simulink model "sampleModel186"  (Simulink 9.1)
settings: Solver=VariableStepAuto  StartTime=0.0  StopTime=10.0  RelTol=1e-3
undefined symbols (not defined in the file): DiscIntNeverNeededParam, Newton, Raphson
libraries: simulink x39
(part 1 of 2)
settings Model: SuppressorTable="22 serialization::archive 11 0 6 0 0 1 8 0 0 0 0 6 0 0 1 0 23 sampleModel186/cfblk100 0 6 0 0 2 8 0 0 0 0 6 41 Simulink:DataType:WarningOverFlowDetected 0 0 0 6 0  0  0 0 0 0 8 20160608 0 0 0 15 23 17 0 1 40 SimulinkFixedPoint:util:Overflowoccurred 0 0 0  0  8 20160608 0 15 23 17 0 1"  Creator=DELL  LastModifiedBy=DELL
settings DataIOCC: SaveFormat=Dataset
settings OptimizationCC: LifeSpan=auto
settings DebuggingCC: UnderspecifiedInitializationDetection=Simplified  MergeDetectMultiDrivingBlocksExec=error  SFUnexpectedBacktrackingDiag=error  SFNoUnconditionalDefaultTransitionDiag=error  SFExecutionAtInitializationDiag=warning
settings HardwareCC: ProdBitPerPointer=64  ProdBitPerSizeT=64  ProdBitPerPtrDiffT=64  ProdLargestAtomicFloat=Float  ProdIntDivRoundTo=Zero  ProdEndianess=LittleEndian  ProdWordSize=64  ProdHWDeviceType=Intel->x86-64 (Windows64)
settings ModelReferenceCC: PropagateSignalLabelsOutOfModel=on
settings CodeAppCC: StateflowObjectComments=off
settings GRTTargetCC: TargetLangStandard=C99 (ISO)  CombineOutputUpdateFcns=on  GRTInterface=off
settings ConfigComp: CovMetricSettings=dwe  CovHtmlReporting=off  CovSaveCumulativeToWorkspaceVar=off  CovSaveSingleToWorkspaceVar=off  CovExternalEMLEnable=on

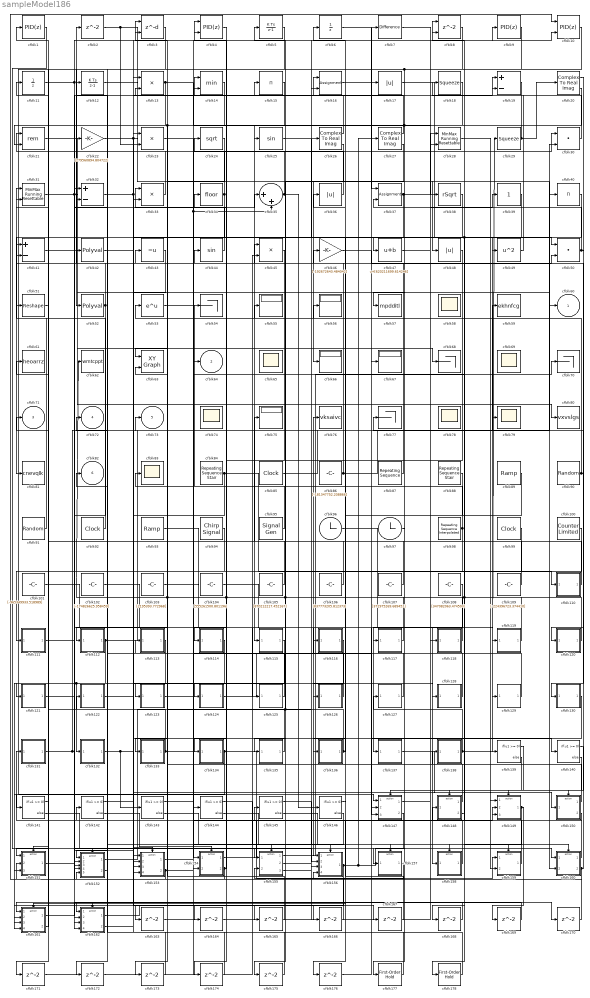
== system sampleModel186 ==
  cfblk1 : simulink/Continuous/PID Controller  Controller=PID  TimeDomain=Discrete-time  SampleTime=1  IntegratorMethod=Forward Euler  FilterMethod=Forward Euler  Form=Parallel  UseFilter=on  ControllerParametersSource=internal  P=1  I=1  D=0  N=100  InitialConditionSource=internal  InitialConditionForIntegrator=0  InitialConditionForFilter=0  ExternalReset=none  LimitOutput=off  UpperSaturationLimit=inf  LowerSaturationLimit=-inf  LinearizeAsGain=off  AntiWindupMode=none  Kb=1  TrackingMode=off  Kt=1  PParamMin=[]  PParamMax=[]  IParamMin=[]  IParamMax=[]  DParamMin=[]  DParamMax=[]  NParamMin=[]  NParamMax=[]  KbParamMin=[]  KbParamMax=[]  KtParamMin=[]  KtParamMax=[]  POutMin=[]  POutMax=[]  IOutMin=[]  IOutMax=[]  DOutMin=[]  DOutMax=[]  NOutMin=[]  NOutMax=[]  KbOutMin=[]  KbOutMax=[]  KtOutMin=[]  KtOutMax=[]  IntegratorOutMin=[]  IntegratorOutMax=[]  FilterOutMin=[]  FilterOutMax=[]  SumOutMin=[]  SumOutMax=[]  SumI1OutMin=[]  SumI1OutMax=[]  SumI2OutMin=[]  SumI2OutMax=[]  SumI3OutMin=[]  SumI3OutMax=[]  SumDOutMin=[]  SumDOutMax=[]  SaturationOutMin=[]  SaturationOutMax=[]  IntegratorContinuousStateAttributes=''  IntegratorStateMustResolveToSignalObject=off  IntegratorRTWStateStorageClass=Auto  FilterContinuousStateAttributes=''  FilterStateMustResolveToSignalObject=off  FilterRTWStateStorageClass=Auto  DifferentiatorICPrevScaledInput=0  DifferentiatorOutMin=[]  DifferentiatorOutMax=[]  FilterDiffOutCoefMin=[]  FilterDiffOutCoefMax=[]  SumDenOutMin=[]  SumDenOutMax=[]  SumNumOutMin=[]  SumNumOutMax=[]  ReciprocalOutMin=[]  ReciprocalOutMax=[]  DivideOutMin=[]  DivideOutMax=[]  TunerSelectOption=Transfer Function Based (PID Tuner App)
  cfblk10 : simulink/Continuous/PID Controller (2DOF)  Controller=PID  TimeDomain=Discrete-time  SampleTime=1  IntegratorMethod=Forward Euler  FilterMethod=Forward Euler  Form=Parallel  UseFilter=on  ControllerParametersSource=internal  P=1  I=1  D=0  N=100  b=1  c=1  InitialConditionSource=internal  InitialConditionForIntegrator=0  InitialConditionForFilter=0  ExternalReset=none  LimitOutput=off  UpperSaturationLimit=inf  LowerSaturationLimit=-inf  LinearizeAsGain=off  AntiWindupMode=none  Kb=1  TrackingMode=off  Kt=1  PParamMin=[]  PParamMax=[]  IParamMin=[]  IParamMax=[]  DParamMin=[]  DParamMax=[]  NParamMin=[]  NParamMax=[]  bParamMin=[]  bParamMax=[]  cParamMin=[]  cParamMax=[]  KbParamMin=[]  KbParamMax=[]  KtParamMin=[]  KtParamMax=[]  POutMin=[]  POutMax=[]  IOutMin=[]  IOutMax=[]  DOutMin=[]  DOutMax=[]  NOutMin=[]  NOutMax=[]  bOutMin=[]  bOutMax=[]  cOutMin=[]  cOutMax=[]  KbOutMin=[]  KbOutMax=[]  KtOutMin=[]  KtOutMax=[]  IntegratorOutMin=[]  IntegratorOutMax=[]  FilterOutMin=[]  FilterOutMax=[]  SumOutMin=[]  SumOutMax=[]  Sum1OutMin=[]  Sum1OutMax=[]  Sum2OutMin=[]  Sum2OutMax=[]  Sum3OutMin=[]  Sum3OutMax=[]  SumI1OutMin=[]  SumI1OutMax=[]  SumI2OutMin=[]  SumI2OutMax=[]  SumI3OutMin=[]  SumI3OutMax=[]  SumDOutMin=[]  SumDOutMax=[]  SaturationOutMin=[]  SaturationOutMax=[]  IntegratorContinuousStateAttributes=''  IntegratorStateMustResolveToSignalObject=off  IntegratorRTWStateStorageClass=Auto  FilterContinuousStateAttributes=''  FilterStateMustResolveToSignalObject=off  FilterRTWStateStorageClass=Auto  DifferentiatorICPrevScaledInput=0  DifferentiatorOutMin=[]  DifferentiatorOutMax=[]  FilterDiffOutCoefMin=[]  FilterDiffOutCoefMax=[]  SumDenOutMin=[]  SumDenOutMax=[]  SumNumOutMin=[]  SumNumOutMax=[]  ReciprocalOutMin=[]  ReciprocalOutMax=[]  DivideOutMin=[]  DivideOutMax=[]  TunerSelectOption=Transfer Function Based (PID Tuner App)
  cfblk100 : simulink/Sources/Counter Limited  uplimit=[470.000000]  tsamp=-1
  cfblk101 : Constant  Value=[-965349933.518989]  SampleTime=1
  cfblk102 : Constant  Value=[-174826625.958459]  SampleTime=1
  cfblk103 : Constant  Value=[2195393.772968]  SampleTime=1
  cfblk104 : Constant  Value=[555261500.801196]  SampleTime=1
  cfblk105 : Constant  Value=[870212217.452167]  SampleTime=1
  cfblk106 : Constant  Value=[837773205.812373]  SampleTime=1
  cfblk107 : Constant  Value=[371975269.689451]  SampleTime=1
  cfblk108 : Constant  Value=[347082063.474503]  SampleTime=1
  cfblk109 : Constant  Value=[-224396723.374410]  SampleTime=1
  cfblk11 : UnitDelay
  cfblk110 : Subsystem
  cfblk111 : Subsystem
  cfblk112 : Subsystem
  cfblk113 : Subsystem
  cfblk114 : Subsystem
  cfblk115 : Subsystem
  cfblk116 : Subsystem
  cfblk117 : Subsystem
  cfblk118 : Subsystem
  cfblk119 : Subsystem
  cfblk12 : DiscreteIntegrator  ICPrevOutput=DiscIntNeverNeededParam  ICPrevScaledInput=DiscIntNeverNeededParam
  cfblk120 : Subsystem
  cfblk121 : Subsystem
  cfblk122 : Subsystem
  cfblk123 : Subsystem
  cfblk124 : Subsystem
  cfblk125 : Subsystem
  cfblk126 : Subsystem
  cfblk127 : Subsystem
  cfblk128 : Subsystem
  cfblk129 : Subsystem
  cfblk13 : Product
  cfblk130 : Subsystem
  cfblk131 : Subsystem
  cfblk132 : Subsystem
  cfblk133 : Subsystem
  cfblk134 : Subsystem
  cfblk135 : Subsystem
  cfblk136 : Subsystem
  cfblk137 : Subsystem
  cfblk138 : Subsystem
  cfblk{139..146} (8 alike) : If  IfExpression=u1 >= 0  SampleTime=1
  cfblk14 : MinMax  Inputs=2
  cfblk147 : Subsystem  TreatAsAtomicUnit=on
  cfblk148 : Subsystem  TreatAsAtomicUnit=on
  cfblk149 : Subsystem  TreatAsAtomicUnit=on
  cfblk15 : Product  Inputs=*
  cfblk150 : Subsystem  TreatAsAtomicUnit=on
  cfblk151 : Subsystem  TreatAsAtomicUnit=on
  cfblk152 : Subsystem  TreatAsAtomicUnit=on
  cfblk153 : Subsystem  TreatAsAtomicUnit=on
  cfblk154 : Subsystem  TreatAsAtomicUnit=on
  cfblk155 : Subsystem  TreatAsAtomicUnit=on
  cfblk156 : Subsystem  TreatAsAtomicUnit=on
  cfblk157 : Subsystem  TreatAsAtomicUnit=on
  cfblk158 : Subsystem  TreatAsAtomicUnit=on
  cfblk159 : Subsystem  TreatAsAtomicUnit=on
  cfblk16 : Assignment  DiagnosticForDimensions=Warning  IndexOptions=Index vector (dialog)  Indices=1  OutputSizes=1
  cfblk160 : Subsystem  TreatAsAtomicUnit=on
  cfblk161 : Subsystem  TreatAsAtomicUnit=on
  cfblk162 : Subsystem  TreatAsAtomicUnit=on
  cfblk{2,163..176} (15 alike) : Delay  SampleTime=1
  cfblk17 : Abs
  cfblk177 : simulink/Discrete/First-Order Hold  DisableCoverage=on  Ts=1
      settings: SourceProductName=Simulink  SourceProductBaseCode=SL
  cfblk178 : simulink/Discrete/First-Order Hold  DisableCoverage=on  Ts=1
      settings: SourceProductName=Simulink  SourceProductBaseCode=SL
  cfblk18 : Squeeze
  cfblk19 : Sum  Inputs=+-
  cfblk20 : ComplexToRealImag
  cfblk21 : Math  Operator=rem  SaturateOnIntegerOverflow=on
  cfblk22 : Gain  Gain=[279560894.804722]
  cfblk23 : Product
  cfblk24 : Sqrt  SaturateOnIntegerOverflow=on
  cfblk25 : Trigonometry
  cfblk26 : ComplexToRealImag
  cfblk27 : ComplexToRealImag
  cfblk28 : simulink/Math Operations/MinMax Running Resettable  Function=min  vinit=0.0
  cfblk29 : Squeeze
  cfblk3 : Delay  DelayLengthSource=Input port  SampleTime=1
      settings: InputPortMap=u0,p1
  cfblk30 : DotProduct  InputSameDT=on  OutDataTypeStr=Inherit: Inherit via internal rule
  cfblk31 : simulink/Math Operations/MinMax Running Resettable  Function=min  vinit=0.0
  cfblk32 : Sum  Inputs=+-
  cfblk33 : Product  Inputs=**
  cfblk34 : Rounding
  cfblk35 : Sum  Inputs=|++
  cfblk36 : Abs
  cfblk37 : Assignment  DiagnosticForDimensions=Warning  IndexOptions=Index vector (dialog)  Indices=1  OutputSizes=1
  cfblk38 : Sqrt  Operator=rSqrt  AlgorithmType=Newton-Raphson  SaturateOnIntegerOverflow=on
  cfblk39 : simulink/Math Operations/Slider Gain  gain=1  low=0  high=2
  cfblk4 : simulink/Continuous/PID Controller (2DOF)  Controller=PID  TimeDomain=Discrete-time  SampleTime=1  IntegratorMethod=Forward Euler  FilterMethod=Forward Euler  Form=Parallel  UseFilter=on  ControllerParametersSource=internal  P=1  I=1  D=0  N=100  b=1  c=1  InitialConditionSource=internal  InitialConditionForIntegrator=0  InitialConditionForFilter=0  ExternalReset=none  LimitOutput=off  UpperSaturationLimit=inf  LowerSaturationLimit=-inf  LinearizeAsGain=off  AntiWindupMode=none  Kb=1  TrackingMode=off  Kt=1  PParamMin=[]  PParamMax=[]  IParamMin=[]  IParamMax=[]  DParamMin=[]  DParamMax=[]  NParamMin=[]  NParamMax=[]  bParamMin=[]  bParamMax=[]  cParamMin=[]  cParamMax=[]  KbParamMin=[]  KbParamMax=[]  KtParamMin=[]  KtParamMax=[]  POutMin=[]  POutMax=[]  IOutMin=[]  IOutMax=[]  DOutMin=[]  DOutMax=[]  NOutMin=[]  NOutMax=[]  bOutMin=[]  bOutMax=[]  cOutMin=[]  cOutMax=[]  KbOutMin=[]  KbOutMax=[]  KtOutMin=[]  KtOutMax=[]  IntegratorOutMin=[]  IntegratorOutMax=[]  FilterOutMin=[]  FilterOutMax=[]  SumOutMin=[]  SumOutMax=[]  Sum1OutMin=[]  Sum1OutMax=[]  Sum2OutMin=[]  Sum2OutMax=[]  Sum3OutMin=[]  Sum3OutMax=[]  SumI1OutMin=[]  SumI1OutMax=[]  SumI2OutMin=[]  SumI2OutMax=[]  SumI3OutMin=[]  SumI3OutMax=[]  SumDOutMin=[]  SumDOutMax=[]  SaturationOutMin=[]  SaturationOutMax=[]  IntegratorContinuousStateAttributes=''  IntegratorStateMustResolveToSignalObject=off  IntegratorRTWStateStorageClass=Auto  FilterContinuousStateAttributes=''  FilterStateMustResolveToSignalObject=off  FilterRTWStateStorageClass=Auto  DifferentiatorICPrevScaledInput=0  DifferentiatorOutMin=[]  DifferentiatorOutMax=[]  FilterDiffOutCoefMin=[]  FilterDiffOutCoefMax=[]  SumDenOutMin=[]  SumDenOutMax=[]  SumNumOutMin=[]  SumNumOutMax=[]  ReciprocalOutMin=[]  ReciprocalOutMax=[]  DivideOutMin=[]  DivideOutMax=[]  TunerSelectOption=Transfer Function Based (PID Tuner App)
  cfblk40 : Product  Inputs=*
  cfblk41 : Sum  Inputs=+-
  cfblk42 : Polyval  Coefs=[ +2.081618890e-019, -1.441693666e-014, +4.719686976e-010, -8.536869453e-006, +1.621573104e-001, -8.087801117e+001 ]
  cfblk43 : UnaryMinus
  cfblk44 : Trigonometry
  cfblk45 : Product  Inputs=**
  cfblk46 : Gain  Gain=[-192672643.484042]
  cfblk47 : Bias  Bias=[620211699.614246]
  cfblk48 : Abs
  cfblk49 : Math  Operator=square  SaturateOnIntegerOverflow=on
  cfblk5 : DiscreteIntegrator  ICPrevOutput=DiscIntNeverNeededParam  ICPrevScaledInput=DiscIntNeverNeededParam
  cfblk50 : DotProduct  InputSameDT=on  OutDataTypeStr=Inherit: Inherit via internal rule
  cfblk51 : Reshape
  cfblk52 : Polyval  Coefs=[ +2.081618890e-019, -1.441693666e-014, +4.719686976e-010, -8.536869453e-006, +1.621573104e-001, -8.087801117e+001 ]
  cfblk53 : Math  SaturateOnIntegerOverflow=on
  cfblk{54,68,70,77} (4 alike) : Terminator
  cfblk{55..56,66..67,75} (5 alike) : Display
  cfblk57 : ToWorkspace  VariableName=mpdditl  SaveFormat=Timeseries  SampleTime=-1
  cfblk{58,65,69,74,78..79,83} (7 alike) : Scope
      cfblk58 settings: Floating=on
      cfblk65 settings: Floating=on
      cfblk69 settings: Floating=on
      cfblk74 settings: Floating=on
      cfblk78 settings: Floating=on
  cfblk59 : ToWorkspace  VariableName=ekhnfcg  SaveFormat=Timeseries  SampleTime=-1
  cfblk6 : UnitDelay
  cfblk61 : ToWorkspace  VariableName=heoarrz  SaveFormat=Timeseries  SampleTime=-1
  cfblk62 : ToWorkspace  VariableName=wmtcppt  SaveFormat=Timeseries  SampleTime=-1
  cfblk63 : simulink/Sinks/XY Graph  xmin=-1  xmax=1  ymin=-1  ymax=1  st=-1
  cfblk7 : simulink/Discrete/Difference  ICPrevInput=0.0  OutMin=[]  OutMax=[]  OutDataTypeStr=Inherit: Inherit via back propagation  OutDataType=fixdt(1, 16)  OutScaling=2^-10  DoSatur=off
  cfblk76 : ToWorkspace  VariableName=vksaivc  SaveFormat=Timeseries  SampleTime=-1
  cfblk8 : Delay  ShowEnablePort=on  SampleTime=1
      settings: InputPortMap=u0,e6
  cfblk80 : ToWorkspace  VariableName=vxvslgs  SaveFormat=Timeseries  SampleTime=-1
  cfblk81 : ToWorkspace  VariableName=cnevqlk  SaveFormat=Timeseries  SampleTime=-1
  cfblk84 : simulink/Sources/Repeating Sequence Stair  OutValues=[-951012836.376546, -301150496.338578]  tsamp=-1  OutMin=[]  OutMax=[]  OutDataTypeStr=double  OutputDataTypeScalingMode=double  OutDataType=fixdt(0,8)  ConRadixGroup=Best Precision: Vector-wise  OutScaling=2^-12
  cfblk85 : DigitalClock
  cfblk86 : Constant  Value=[-181347752.208866]  SampleTime=1
  cfblk87 : simulink/Sources/Repeating Sequence  rep_seq_t=[0 2]  rep_seq_y=[440494450.888145, 19517650.074052]
  cfblk88 : simulink/Sources/Repeating Sequence Stair  OutValues=[252287752.212713, -649877738.569084]  tsamp=-1  OutMin=[]  OutMax=[]  OutDataTypeStr=double  OutputDataTypeScalingMode=double  OutDataType=fixdt(0,8)  ConRadixGroup=Best Precision: Vector-wise  OutScaling=2^-12
  cfblk89 : simulink/Sources/Ramp  slope=[7648.383013]  start=[49.860046]  InitialOutput=[-317458.336666]
  cfblk9 : simulink/Continuous/PID Controller  Controller=PID  TimeDomain=Discrete-time  SampleTime=1  IntegratorMethod=Forward Euler  FilterMethod=Forward Euler  Form=Parallel  UseFilter=on  ControllerParametersSource=internal  P=1  I=1  D=0  N=100  InitialConditionSource=internal  InitialConditionForIntegrator=0  InitialConditionForFilter=0  ExternalReset=none  LimitOutput=off  UpperSaturationLimit=inf  LowerSaturationLimit=-inf  LinearizeAsGain=off  AntiWindupMode=none  Kb=1  TrackingMode=off  Kt=1  PParamMin=[]  PParamMax=[]  IParamMin=[]  IParamMax=[]  DParamMin=[]  DParamMax=[]  NParamMin=[]  NParamMax=[]  KbParamMin=[]  KbParamMax=[]  KtParamMin=[]  KtParamMax=[]  POutMin=[]  POutMax=[]  IOutMin=[]  IOutMax=[]  DOutMin=[]  DOutMax=[]  NOutMin=[]  NOutMax=[]  KbOutMin=[]  KbOutMax=[]  KtOutMin=[]  KtOutMax=[]  IntegratorOutMin=[]  IntegratorOutMax=[]  FilterOutMin=[]  FilterOutMax=[]  SumOutMin=[]  SumOutMax=[]  SumI1OutMin=[]  SumI1OutMax=[]  SumI2OutMin=[]  SumI2OutMax=[]  SumI3OutMin=[]  SumI3OutMax=[]  SumDOutMin=[]  SumDOutMax=[]  SaturationOutMin=[]  SaturationOutMax=[]  IntegratorContinuousStateAttributes=''  IntegratorStateMustResolveToSignalObject=off  IntegratorRTWStateStorageClass=Auto  FilterContinuousStateAttributes=''  FilterStateMustResolveToSignalObject=off  FilterRTWStateStorageClass=Auto  DifferentiatorICPrevScaledInput=0  DifferentiatorOutMin=[]  DifferentiatorOutMax=[]  FilterDiffOutCoefMin=[]  FilterDiffOutCoefMax=[]  SumDenOutMin=[]  SumDenOutMax=[]  SumNumOutMin=[]  SumNumOutMax=[]  ReciprocalOutMin=[]  ReciprocalOutMax=[]  DivideOutMin=[]  DivideOutMax=[]  TunerSelectOption=Transfer Function Based (PID Tuner App)
  cfblk90 : RandomNumber  Mean=[38383.504717]  Variance=[46527.170956]  Seed=[481409235.000000]  SampleTime=0.1
  cfblk91 : RandomNumber  Mean=[-57930.765169]  Variance=[93296.523192]  Seed=[604567942.000000]  SampleTime=0.1
  cfblk92 : DigitalClock
  cfblk93 : simulink/Sources/Ramp  slope=[805.402797]  start=[19.130150]  InitialOutput=[280438.468677]
  cfblk94 : simulink/Sources/Chirp Signal  f1=[-292046844.976813]  T=[-444072076.223065]  f2=[-648078448.170480]
  cfblk95 : SignalGenerator  Amplitude=[-110026774.580728]
  cfblk96 : Clock
  cfblk97 : Clock
  cfblk98 : simulink/Sources/Repeating Sequence Interpolated  OutValues=[-130836063.192327, 223313554.665259, -659778868.713167, 244454041.153535, 249774118.930075]  TimeValues=[0 0.1 0.5 0.6 1].'  LookUpMeth=Use Input Nearest  tsamp=0.01  OutMin=[]  OutMax=[]  OutDataTypeStr=double  OutputDataTypeScalingMode=double  OutDataType=fixdt(0,8)  OutScaling=2^-10
  cfblk99 : DigitalClock
  cfblk60 : Outport
  cfblk64 : Outport  Port=2
  cfblk71 : Outport  Port=3
  cfblk72 : Outport  Port=4
  cfblk73 : Outport  Port=5
  cfblk82 : Outport  Port=6
  wires:
  cfblk44/1 -> cfblk33/1
  cfblk113/1(cfblk2) -> cfblk132/1(cfblk1), cfblk161/4(cfblk15)
  cfblk21/1 -> cfblk80/1
  cfblk131/1(cfblk2) -> cfblk73/1, cfblk153/4(cfblk11)
  cfblk3/1 -> cfblk147/1(cfblk1)
  cfblk40/1 -> cfblk81/1
  cfblk148/1(cfblk2) -> cfblk112/1(cfblk1)
  cfblk20/1 -> cfblk77/1
  cfblk84/1 -> cfblk110/1(cfblk1), cfblk153/3(cfblk10)
  cfblk155/1(cfblk2) -> cfblk70/1
  cfblk12/1 -> cfblk66/1
  cfblk119/1(cfblk2) -> cfblk43/1, cfblk8/2
  cfblk110/1(cfblk2) -> cfblk46/1
  cfblk96/1 -> cfblk158/1(cfblk1)
  cfblk1/1 -> cfblk159/1(cfblk1)
  cfblk138/1(cfblk2) -> cfblk29/1, cfblk127/1(cfblk1)
  cfblk95/1 -> cfblk54/1
  cfblk23/1 -> cfblk154/1(cfblk1)
  cfblk2/1 -> cfblk48/1, cfblk23/2
  cfblk18/1 -> cfblk114/1(cfblk1)
  cfblk103/1 -> cfblk156/1(cfblk1)
  cfblk109/1 -> cfblk36/1
  cfblk130/1(cfblk2) -> cfblk147/2(cfblk10)
  cfblk149/1(cfblk2) -> cfblk168/1, cfblk169/1
  cfblk41/1 -> cfblk68/1
  cfblk101/1 -> cfblk144/1
  cfblk156/1(cfblk2) -> cfblk160/1(cfblk1), cfblk27/1, cfblk161/2(cfblk13)
  cfblk24/1 -> cfblk63/1
  cfblk134/1(cfblk2) -> cfblk156/2(cfblk11), cfblk161/3(cfblk14)
  cfblk136/1(cfblk2) -> cfblk113/1(cfblk1), cfblk55/1, cfblk6/1
  cfblk114/1(cfblk2) -> cfblk124/1(cfblk1)
  cfblk17/1 -> cfblk129/1(cfblk1)
  cfblk158/1(cfblk2) -> cfblk131/1(cfblk1)
  cfblk15/1 -> cfblk115/1(cfblk1)
  cfblk34/1 -> cfblk24/1, cfblk171/1
  cfblk29/1 -> cfblk25/1, cfblk20/1
  cfblk47/1 -> cfblk39/1
  cfblk124/1(cfblk2) -> cfblk67/1
  cfblk107/1 -> cfblk75/1
  cfblk154/1(cfblk2) -> cfblk148/1(cfblk1)
  cfblk137/1(cfblk2) -> cfblk159/2(cfblk12)
  cfblk117/1(cfblk2) -> cfblk14/1, cfblk42/1
  cfblk148/2(cfblk9) -> cfblk64/1
  cfblk50/1 -> cfblk120/1(cfblk1), cfblk37/2
  cfblk108/1 -> cfblk137/1(cfblk1)
  cfblk128/1(cfblk2) -> cfblk5/1
  cfblk10/1 -> cfblk52/1
  cfblk30/1 -> cfblk18/1
  cfblk28/1 -> cfblk50/1
  cfblk120/1(cfblk2) -> cfblk62/1, cfblk63/2, cfblk45/1
  cfblk87/1 -> cfblk2/1
  cfblk99/1 -> cfblk155/1(cfblk1)
  cfblk91/1 -> cfblk31/1
  cfblk42/1 -> cfblk128/1(cfblk1)
  cfblk16/1 -> cfblk17/1
  cfblk48/1 -> cfblk135/1(cfblk1)
  cfblk39/1 -> cfblk163/1, cfblk178/1
  cfblk159/1(cfblk2) -> cfblk82/1
  cfblk115/1(cfblk2) -> cfblk123/1(cfblk1)
  cfblk160/1(cfblk2) -> cfblk138/1(cfblk1)
  cfblk6/1 -> cfblk37/1
  cfblk150/1(cfblk2) -> cfblk34/1
  cfblk94/1 -> cfblk141/1
  cfblk126/1(cfblk2) -> cfblk76/1
  cfblk102/1 -> cfblk125/1(cfblk1)
  cfblk98/1 -> cfblk111/1(cfblk1), cfblk3/2
  cfblk106/1 -> cfblk71/1
  cfblk153/1(cfblk2) -> cfblk30/1
  cfblk32/1 -> cfblk8/1, cfblk49/1
  cfblk105/1 -> cfblk51/1
  cfblk147/1(cfblk2) -> cfblk118/1(cfblk1)
  cfblk133/1(cfblk2) -> cfblk11/1, cfblk116/1(cfblk1)
  cfblk118/1(cfblk2) -> cfblk56/1
  cfblk152/1(cfblk2) -> cfblk26/1
  cfblk90/1 -> cfblk130/1(cfblk1), cfblk53/1
  cfblk51/1 -> cfblk151/1(cfblk1)
  cfblk112/1(cfblk2) -> cfblk59/1, cfblk151/3(cfblk11)
  cfblk157/1(cfblk2) -> cfblk156/4(cfblk13)
  cfblk135/1(cfblk2) -> cfblk83/1
  cfblk111/1(cfblk2) -> cfblk119/1(cfblk1)
  cfblk27/1 -> cfblk16/1
  cfblk53/1 -> cfblk19/1
  cfblk97/1 -> cfblk157/1(cfblk1)
  cfblk104/1 -> cfblk139/1
  cfblk37/1 -> cfblk149/1(cfblk1), cfblk162/3(cfblk14)
  cfblk25/1 -> cfblk47/1
  cfblk8/1 -> cfblk117/1(cfblk1), cfblk172/1
  cfblk22/1 -> cfblk60/1, cfblk140/1
  cfblk45/1 -> cfblk134/1(cfblk1)
  cfblk155/2(cfblk6) -> cfblk16/2
  cfblk31/1 -> cfblk160/2(cfblk6), cfblk15/1
  cfblk46/1 -> cfblk50/2
  cfblk43/1 -> cfblk153/2(cfblk9)
  cfblk5/1 -> cfblk41/1
  cfblk85/1 -> cfblk30/2
  cfblk35/1 -> cfblk21/1, cfblk146/1
  cfblk153/2(cfblk12) -> cfblk10/1, cfblk149/3(cfblk11)
  cfblk127/1(cfblk2) -> cfblk72/1
  cfblk155/3(cfblk7) -> cfblk10/2
  cfblk36/1 -> cfblk14/2
  cfblk9/1 -> cfblk152/1(cfblk1)
  cfblk86/1 -> cfblk40/1, cfblk1/1
  cfblk19/1 -> cfblk57/1, cfblk173/1
  cfblk14/1 -> cfblk133/1(cfblk1), cfblk121/1(cfblk1)
  cfblk100/1 -> cfblk162/2(cfblk13)
  cfblk7/1 -> cfblk38/1
  cfblk151/1(cfblk2) -> cfblk79/1
  cfblk33/1 -> cfblk22/1
  cfblk116/1(cfblk2) -> cfblk126/1(cfblk1)
  cfblk129/1(cfblk2) -> cfblk4/1
  cfblk160/2(cfblk7) -> cfblk44/1, cfblk152/5(cfblk16)
  cfblk92/1 -> cfblk31/2
  cfblk52/1 -> cfblk41/2, cfblk162/4(cfblk15)
  cfblk13/1 -> cfblk21/2, cfblk28/2
  cfblk132/1(cfblk2) -> cfblk150/1(cfblk1), cfblk143/1
  cfblk152/2(cfblk17) -> cfblk122/1(cfblk1)
  cfblk147/2(cfblk12) -> cfblk152/3(cfblk14)
  cfblk93/1 -> cfblk147/3(cfblk11)
  cfblk89/1 -> cfblk136/1(cfblk1)
  cfblk123/1(cfblk2) -> cfblk9/1, cfblk35/2
  cfblk11/1 -> cfblk152/4(cfblk15), cfblk3/1
  cfblk26/1 -> cfblk4/2
  cfblk125/1(cfblk2) -> cfblk12/1
  cfblk150/2(cfblk14) -> cfblk149/2(cfblk10)
  cfblk161/2(cfblk16) -> cfblk61/1
  cfblk162/2(cfblk16) -> cfblk33/2
  cfblk154/2(cfblk15) -> cfblk13/2, cfblk151/2(cfblk10)
  cfblk121/1(cfblk2) -> cfblk35/1
  cfblk49/1 -> cfblk19/2
  cfblk139/1 -> cfblk147/Action
  cfblk139/2 -> cfblk148/Action
  cfblk140/1 -> cfblk149/Action
  cfblk140/2 -> cfblk150/Action
  cfblk141/1 -> cfblk151/Action
  cfblk141/2 -> cfblk152/Action
  cfblk142/1 -> cfblk153/Action
  cfblk142/2 -> cfblk154/Action
  cfblk143/1 -> cfblk155/Action
  cfblk143/2 -> cfblk156/Action
  cfblk144/1 -> cfblk157/Action
  cfblk144/2 -> cfblk158/Action
  cfblk145/1 -> cfblk159/Action
  cfblk145/2 -> cfblk160/Action
  cfblk146/1 -> cfblk161/Action
  cfblk146/2 -> cfblk162/Action
  cfblk163/1 -> cfblk28/1
  cfblk4/1 -> cfblk164/1
  cfblk164/1 -> cfblk156/3(cfblk12)
  cfblk26/2 -> cfblk165/1
  cfblk165/1 -> cfblk13/1
  cfblk122/1(cfblk2) -> cfblk166/1
  cfblk166/1 -> cfblk155/2(cfblk5)
  cfblk162/1(cfblk2) -> cfblk167/1
  cfblk167/1 -> cfblk145/1
  cfblk168/1 -> cfblk162/1(cfblk1)
  cfblk169/1 -> cfblk161/1(cfblk1)
  cfblk161/1(cfblk2) -> cfblk170/1
  cfblk170/1 -> cfblk152/2(cfblk13)
  cfblk171/1 -> cfblk154/2(cfblk14)
  cfblk172/1 -> cfblk45/2
  cfblk173/1 -> cfblk23/1
  cfblk20/2 -> cfblk174/1
  cfblk174/1 -> cfblk142/1
  cfblk27/2 -> cfblk175/1
  cfblk175/1 -> cfblk153/1(cfblk1)
  cfblk38/1 -> cfblk176/1
  cfblk176/1 -> cfblk7/1
  cfblk88/1 -> cfblk177/1
  cfblk177/1 -> cfblk32/1
  cfblk178/1 -> cfblk32/2

== system sampleModel186/cfblk110 ==
  cfblk1 : Inport
  cfblk2 : Outport
  wires:
  cfblk1/1 -> cfblk2/1

== system sampleModel186/cfblk111 ==
  cfblk1 : Inport
  cfblk2 : Outport
  wires:
  cfblk1/1 -> cfblk2/1

== system sampleModel186/cfblk112 ==
  cfblk1 : Inport
  cfblk2 : Outport
  wires:
  cfblk1/1 -> cfblk2/1

== system sampleModel186/cfblk113 ==
  cfblk1 : Inport
  cfblk2 : Outport
  wires:
  cfblk1/1 -> cfblk2/1

== system sampleModel186/cfblk114 ==
  cfblk1 : Inport
  cfblk2 : Outport
  wires:
  cfblk1/1 -> cfblk2/1

== system sampleModel186/cfblk115 ==
  cfblk1 : Inport
  cfblk2 : Outport
  wires:
  cfblk1/1 -> cfblk2/1

== system sampleModel186/cfblk116 ==
  cfblk1 : Inport
  cfblk2 : Outport
  wires:
  cfblk1/1 -> cfblk2/1

== system sampleModel186/cfblk117 ==
  cfblk1 : Inport
  cfblk2 : Outport
  wires:
  cfblk1/1 -> cfblk2/1

== system sampleModel186/cfblk118 ==
  cfblk1 : Inport
  cfblk2 : Outport
  wires:
  cfblk1/1 -> cfblk2/1

== system sampleModel186/cfblk119 ==
  cfblk1 : Inport
  cfblk2 : Outport
  wires:
  cfblk1/1 -> cfblk2/1

== system sampleModel186/cfblk120 ==
  cfblk1 : Inport
  cfblk2 : Outport
  wires:
  cfblk1/1 -> cfblk2/1

== system sampleModel186/cfblk121 ==
  cfblk1 : Inport
  cfblk2 : Outport
  wires:
  cfblk1/1 -> cfblk2/1

== system sampleModel186/cfblk122 ==
  cfblk1 : Inport
  cfblk2 : Outport
  wires:
  cfblk1/1 -> cfblk2/1

== system sampleModel186/cfblk123 ==
  cfblk1 : Inport
  cfblk2 : Outport
  wires:
  cfblk1/1 -> cfblk2/1

== system sampleModel186/cfblk124 ==
  cfblk1 : Inport
  cfblk2 : Outport
  wires:
  cfblk1/1 -> cfblk2/1

== system sampleModel186/cfblk125 ==
  cfblk1 : Inport
  cfblk2 : Outport
  wires:
  cfblk1/1 -> cfblk2/1

== system sampleModel186/cfblk126 ==
  cfblk1 : Inport
  cfblk2 : Outport
  wires:
  cfblk1/1 -> cfblk2/1

== system sampleModel186/cfblk127 ==
  cfblk1 : Inport
  cfblk2 : Outport
  wires:
  cfblk1/1 -> cfblk2/1

== system sampleModel186/cfblk128 ==
  cfblk1 : Inport
  cfblk2 : Outport
  wires:
  cfblk1/1 -> cfblk2/1

== system sampleModel186/cfblk129 ==
  cfblk1 : Inport
  cfblk2 : Outport
  wires:
  cfblk1/1 -> cfblk2/1

== system sampleModel186/cfblk130 ==
  cfblk1 : Inport
  cfblk2 : Outport
  wires:
  cfblk1/1 -> cfblk2/1

== system sampleModel186/cfblk131 ==
  cfblk1 : Inport
  cfblk2 : Outport
  wires:
  cfblk1/1 -> cfblk2/1

== system sampleModel186/cfblk132 ==
  cfblk1 : Inport
  cfblk2 : Outport
  wires:
  cfblk1/1 -> cfblk2/1

== system sampleModel186/cfblk133 ==
  cfblk1 : Inport
  cfblk2 : Outport
  wires:
  cfblk1/1 -> cfblk2/1

== system sampleModel186/cfblk134 ==
  cfblk1 : Inport
  cfblk2 : Outport
  wires:
  cfblk1/1 -> cfblk2/1

== system sampleModel186/cfblk135 ==
  cfblk1 : Inport
  cfblk2 : Outport
  wires:
  cfblk1/1 -> cfblk2/1

== system sampleModel186/cfblk136 ==
  cfblk1 : Inport
  cfblk2 : Outport
  wires:
  cfblk1/1 -> cfblk2/1

== system sampleModel186/cfblk137 ==
  cfblk1 : Inport
  cfblk2 : Outport
  wires:
  cfblk1/1 -> cfblk2/1

== system sampleModel186/cfblk138 ==
  cfblk1 : Inport
  cfblk2 : Outport
  wires:
  cfblk1/1 -> cfblk2/1

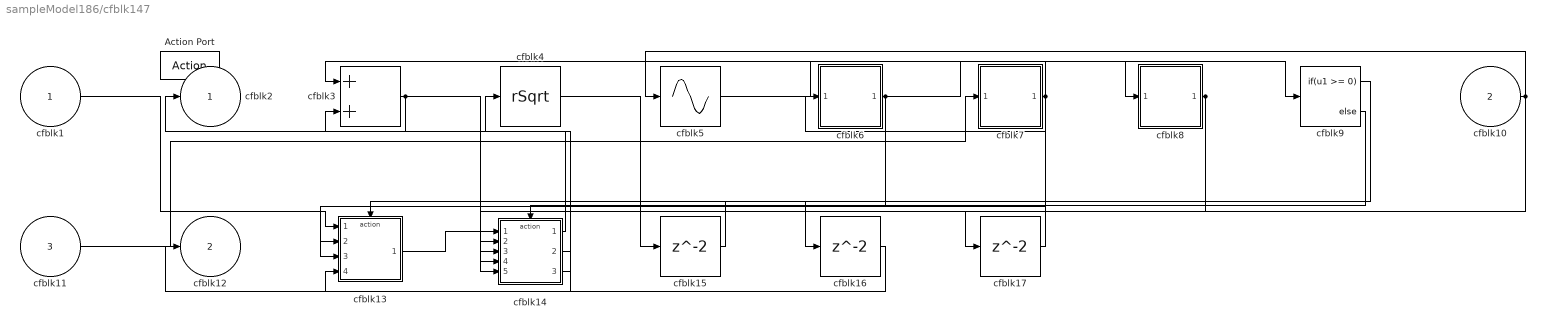
== system sampleModel186/cfblk147 ==
  cfblk1 : Inport
  cfblk10 : Inport  Port=2
  cfblk11 : Inport  Port=3
  Action Port : ActionPort  ActionType=then
  cfblk13 : Subsystem  TreatAsAtomicUnit=on
  cfblk14 : Subsystem  TreatAsAtomicUnit=on
  cfblk15 : Delay
  cfblk16 : Delay
  cfblk17 : Delay
  cfblk3 : Sum
  cfblk4 : Sqrt  Operator=rSqrt  AlgorithmType=Newton-Raphson  SaturateOnIntegerOverflow=on
  cfblk5 : Sin  TimeSource=Use external signal  SampleTime=0
  cfblk6 : Subsystem
  cfblk7 : Subsystem
  cfblk8 : Subsystem
  cfblk9 : If  IfExpression=u1 >= 0  SampleTime=1
  cfblk2 : Outport
  cfblk12 : Outport  Port=2
  wires:
  cfblk3/1 -> cfblk2/1, cfblk16/1
  cfblk11/1 -> cfblk7/1(cfblk1)
  cfblk5/1 -> cfblk9/1
  cfblk6/1(cfblk2) -> cfblk8/1(cfblk1), cfblk13/2(cfblk8)
  cfblk10/1 -> cfblk5/1, cfblk14/3(cfblk10)
  cfblk13/1(cfblk2) -> cfblk14/1(cfblk1)
  cfblk8/1(cfblk2) -> cfblk14/4(cfblk11), cfblk17/1
  cfblk7/1(cfblk2) -> cfblk3/1, cfblk13/3(cfblk9), cfblk14/5(cfblk12)
  cfblk14/1(cfblk2) -> cfblk4/1
  cfblk14/2(cfblk13) -> cfblk12/1
  cfblk14/3(cfblk14) -> cfblk3/2
  cfblk1/1 -> cfblk13/1(cfblk1)
  cfblk9/1 -> cfblk13/Action
  cfblk9/2 -> cfblk14/Action
  cfblk4/1 -> cfblk15/1
  cfblk15/1 -> cfblk14/2(cfblk9)
  cfblk16/1 -> cfblk13/4(cfblk10)
  cfblk17/1 -> cfblk6/1(cfblk1)

== system sampleModel186/cfblk148 ==
  cfblk1 : Inport
  Action Port : ActionPort  ActionType=else
  cfblk10 : Delay
  cfblk3 : Assignment  DiagnosticForDimensions=Warning  IndexOptions=Index vector (dialog)  Indices=1  OutputSizes=1
  cfblk4 : Assignment  DiagnosticForDimensions=Warning  IndexOptions=Index vector (dialog)  Indices=1  OutputSizes=1
  cfblk5 : Gain  Gain=[101234097.543843]
  cfblk6 : Subsystem
  cfblk7 : Subsystem
  cfblk8 : Subsystem
  cfblk2 : Outport
  cfblk9 : Outport  Port=2
  wires:
  cfblk6/1(cfblk2) -> cfblk4/1
  cfblk7/1(cfblk2) -> cfblk8/1(cfblk1)
  cfblk1/1 -> cfblk6/1(cfblk1)
  cfblk5/1 -> cfblk4/2, cfblk7/1(cfblk1), cfblk3/2
  cfblk3/1 -> cfblk2/1
  cfblk8/1(cfblk2) -> cfblk3/1, cfblk10/1
  cfblk4/1 -> cfblk9/1
  cfblk10/1 -> cfblk5/1

== system sampleModel186/cfblk149 ==
  cfblk1 : Inport
  cfblk10 : Inport  Port=2
  cfblk11 : Inport  Port=3
  Action Port : ActionPort  ActionType=then
  cfblk3 : simulink/Discrete/Difference  ICPrevInput=0.0  OutMin=[]  OutMax=[]  OutDataTypeStr=Inherit: Inherit via back propagation  OutDataType=fixdt(1, 16)  OutScaling=2^-10  DoSatur=off
  cfblk4 : DiscreteFilter
  cfblk5 : simulink/Math Operations/Slider Gain  gain=1  low=0  high=2
  cfblk6 : Product
  cfblk7 : Product  Inputs=**
  cfblk8 : Constant  Value=[763231843.033277]  SampleTime=1
  cfblk9 : Subsystem
  cfblk2 : Outport
  wires:
  cfblk10/1 -> cfblk9/1(cfblk1)
  cfblk4/1 -> cfblk7/1
  cfblk8/1 -> cfblk3/1
  cfblk5/1 -> cfblk7/2
  cfblk9/1(cfblk2) -> cfblk4/1
  cfblk3/1 -> cfblk5/1
  cfblk11/1 -> cfblk2/1
  cfblk1/1 -> cfblk6/1
  cfblk7/1 -> cfblk6/2

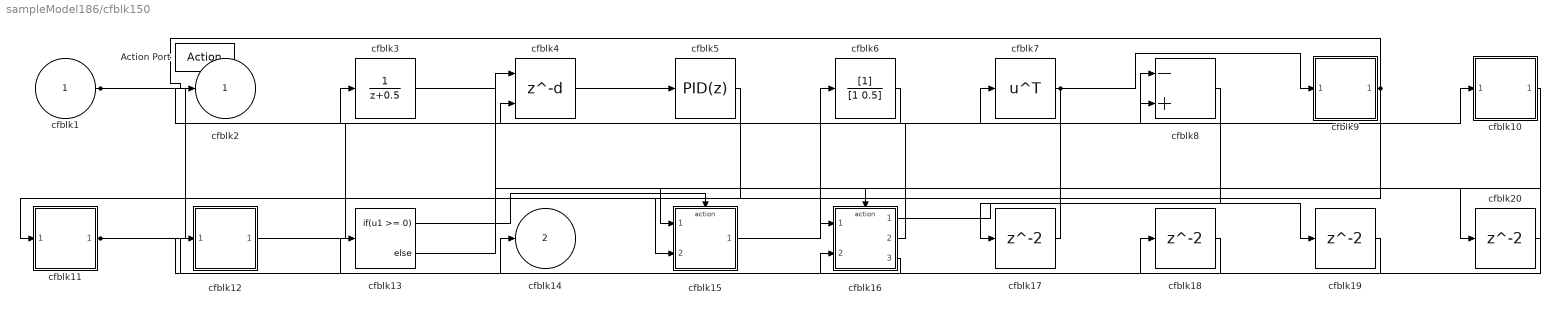
== system sampleModel186/cfblk150 ==
  cfblk1 : Inport
  Action Port : ActionPort  ActionType=else
  cfblk10 : Subsystem
  cfblk11 : Subsystem
  cfblk12 : Subsystem
  cfblk13 : If  IfExpression=u1 >= 0  SampleTime=1
  cfblk15 : Subsystem  TreatAsAtomicUnit=on
  cfblk16 : Subsystem  TreatAsAtomicUnit=on
  cfblk{17..20} (4 alike) : Delay
  cfblk3 : DiscreteTransferFcn
  cfblk4 : Delay  DelayLengthSource=Input port
      settings: InputPortMap=u0,p1
  cfblk5 : simulink/Continuous/PID Controller  Controller=PID  TimeDomain=Discrete-time  SampleTime=-1  IntegratorMethod=Forward Euler  FilterMethod=Forward Euler  Form=Parallel  UseFilter=on  ControllerParametersSource=internal  P=1  I=1  D=0  N=100  InitialConditionSource=internal  InitialConditionForIntegrator=0  InitialConditionForFilter=0  ExternalReset=none  LimitOutput=off  UpperSaturationLimit=inf  LowerSaturationLimit=-inf  LinearizeAsGain=off  AntiWindupMode=none  Kb=1  TrackingMode=off  Kt=1  PParamMin=[]  PParamMax=[]  IParamMin=[]  IParamMax=[]  DParamMin=[]  DParamMax=[]  NParamMin=[]  NParamMax=[]  KbParamMin=[]  KbParamMax=[]  KtParamMin=[]  KtParamMax=[]  POutMin=[]  POutMax=[]  IOutMin=[]  IOutMax=[]  DOutMin=[]  DOutMax=[]  NOutMin=[]  NOutMax=[]  KbOutMin=[]  KbOutMax=[]  KtOutMin=[]  KtOutMax=[]  IntegratorOutMin=[]  IntegratorOutMax=[]  FilterOutMin=[]  FilterOutMax=[]  SumOutMin=[]  SumOutMax=[]  SumI1OutMin=[]  SumI1OutMax=[]  SumI2OutMin=[]  SumI2OutMax=[]  SumI3OutMin=[]  SumI3OutMax=[]  SumDOutMin=[]  SumDOutMax=[]  SaturationOutMin=[]  SaturationOutMax=[]  IntegratorContinuousStateAttributes=''  IntegratorStateMustResolveToSignalObject=off  IntegratorRTWStateStorageClass=Auto  FilterContinuousStateAttributes=''  FilterStateMustResolveToSignalObject=off  FilterRTWStateStorageClass=Auto  DifferentiatorICPrevScaledInput=0  DifferentiatorOutMin=[]  DifferentiatorOutMax=[]  FilterDiffOutCoefMin=[]  FilterDiffOutCoefMax=[]  SumDenOutMin=[]  SumDenOutMax=[]  SumNumOutMin=[]  SumNumOutMax=[]  ReciprocalOutMin=[]  ReciprocalOutMax=[]  DivideOutMin=[]  DivideOutMax=[]  TunerSelectOption=Transfer Function Based (PID Tuner App)
  cfblk6 : DiscreteFilter
  cfblk7 : Math  Operator=transpose  SaturateOnIntegerOverflow=on
  cfblk8 : Sum  Inputs=-+
  cfblk9 : Subsystem
  cfblk2 : Outport
  cfblk14 : Outport  Port=2
  wires:
  cfblk11/1(cfblk2) -> cfblk8/1, cfblk18/1
  cfblk12/1(cfblk2) -> cfblk8/2
  cfblk15/1(cfblk2) -> cfblk6/1
  cfblk4/1 -> cfblk5/1
  cfblk7/1 -> cfblk9/1(cfblk1), cfblk16/1(cfblk1)
  cfblk6/1 -> cfblk4/2
  cfblk10/1(cfblk2) -> cfblk12/1(cfblk1)
  cfblk5/1 -> cfblk11/1(cfblk1)
  cfblk1/1 -> cfblk7/1, cfblk10/1(cfblk1)
  cfblk16/2(cfblk11) -> cfblk3/1
  cfblk16/3(cfblk12) -> cfblk14/1
  cfblk9/1(cfblk2) -> cfblk2/1, cfblk15/2(cfblk15)
  cfblk13/1 -> cfblk15/Action
  cfblk13/2 -> cfblk16/Action
  cfblk8/1 -> cfblk17/1
  cfblk17/1 -> cfblk4/1
  cfblk18/1 -> cfblk16/2(cfblk10)
  cfblk16/1(cfblk2) -> cfblk19/1
  cfblk19/1 -> cfblk13/1
  cfblk3/1 -> cfblk20/1
  cfblk20/1 -> cfblk15/1(cfblk1)

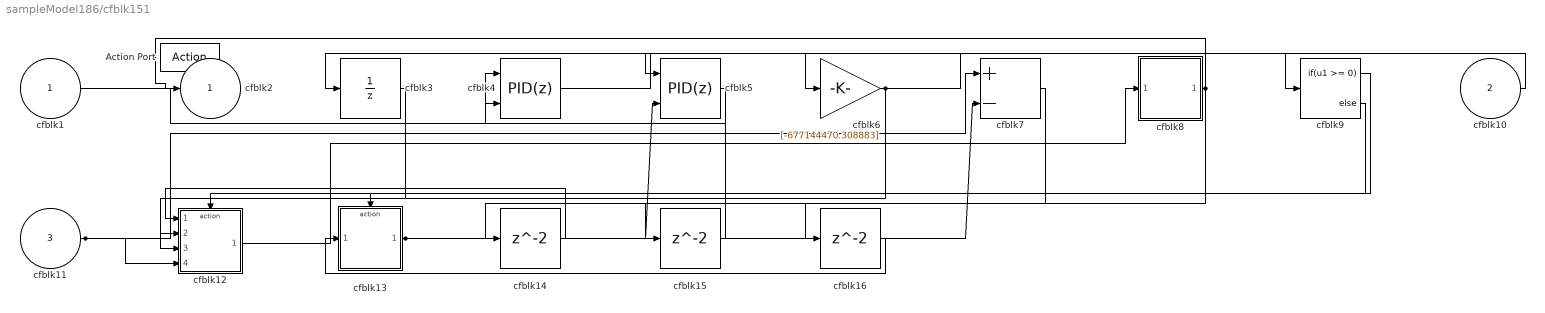
== system sampleModel186/cfblk151 ==
  cfblk1 : Inport
  cfblk10 : Inport  Port=2
  cfblk11 : Inport  Port=3
  Action Port : ActionPort  ActionType=then
  cfblk12 : Subsystem  TreatAsAtomicUnit=on
  cfblk13 : Subsystem  TreatAsAtomicUnit=on
  cfblk14 : Delay
  cfblk15 : Delay
  cfblk16 : Delay
  cfblk3 : UnitDelay  SampleTime=-1
  cfblk4 : simulink/Continuous/PID Controller (2DOF)  Controller=PID  TimeDomain=Discrete-time  SampleTime=-1  IntegratorMethod=Forward Euler  FilterMethod=Forward Euler  Form=Parallel  UseFilter=on  ControllerParametersSource=internal  P=1  I=1  D=0  N=100  b=1  c=1  InitialConditionSource=internal  InitialConditionForIntegrator=0  InitialConditionForFilter=0  ExternalReset=none  LimitOutput=off  UpperSaturationLimit=inf  LowerSaturationLimit=-inf  LinearizeAsGain=off  AntiWindupMode=none  Kb=1  TrackingMode=off  Kt=1  PParamMin=[]  PParamMax=[]  IParamMin=[]  IParamMax=[]  DParamMin=[]  DParamMax=[]  NParamMin=[]  NParamMax=[]  bParamMin=[]  bParamMax=[]  cParamMin=[]  cParamMax=[]  KbParamMin=[]  KbParamMax=[]  KtParamMin=[]  KtParamMax=[]  POutMin=[]  POutMax=[]  IOutMin=[]  IOutMax=[]  DOutMin=[]  DOutMax=[]  NOutMin=[]  NOutMax=[]  bOutMin=[]  bOutMax=[]  cOutMin=[]  cOutMax=[]  KbOutMin=[]  KbOutMax=[]  KtOutMin=[]  KtOutMax=[]  IntegratorOutMin=[]  IntegratorOutMax=[]  FilterOutMin=[]  FilterOutMax=[]  SumOutMin=[]  SumOutMax=[]  Sum1OutMin=[]  Sum1OutMax=[]  Sum2OutMin=[]  Sum2OutMax=[]  Sum3OutMin=[]  Sum3OutMax=[]  SumI1OutMin=[]  SumI1OutMax=[]  SumI2OutMin=[]  SumI2OutMax=[]  SumI3OutMin=[]  SumI3OutMax=[]  SumDOutMin=[]  SumDOutMax=[]  SaturationOutMin=[]  SaturationOutMax=[]  IntegratorContinuousStateAttributes=''  IntegratorStateMustResolveToSignalObject=off  IntegratorRTWStateStorageClass=Auto  FilterContinuousStateAttributes=''  FilterStateMustResolveToSignalObject=off  FilterRTWStateStorageClass=Auto  DifferentiatorICPrevScaledInput=0  DifferentiatorOutMin=[]  DifferentiatorOutMax=[]  FilterDiffOutCoefMin=[]  FilterDiffOutCoefMax=[]  SumDenOutMin=[]  SumDenOutMax=[]  SumNumOutMin=[]  SumNumOutMax=[]  ReciprocalOutMin=[]  ReciprocalOutMax=[]  DivideOutMin=[]  DivideOutMax=[]  TunerSelectOption=Transfer Function Based (PID Tuner App)
  cfblk5 : simulink/Continuous/PID Controller (2DOF)  Controller=PID  TimeDomain=Discrete-time  SampleTime=-1  IntegratorMethod=Forward Euler  FilterMethod=Forward Euler  Form=Parallel  UseFilter=on  ControllerParametersSource=internal  P=1  I=1  D=0  N=100  b=1  c=1  InitialConditionSource=internal  InitialConditionForIntegrator=0  InitialConditionForFilter=0  ExternalReset=none  LimitOutput=off  UpperSaturationLimit=inf  LowerSaturationLimit=-inf  LinearizeAsGain=off  AntiWindupMode=none  Kb=1  TrackingMode=off  Kt=1  PParamMin=[]  PParamMax=[]  IParamMin=[]  IParamMax=[]  DParamMin=[]  DParamMax=[]  NParamMin=[]  NParamMax=[]  bParamMin=[]  bParamMax=[]  cParamMin=[]  cParamMax=[]  KbParamMin=[]  KbParamMax=[]  KtParamMin=[]  KtParamMax=[]  POutMin=[]  POutMax=[]  IOutMin=[]  IOutMax=[]  DOutMin=[]  DOutMax=[]  NOutMin=[]  NOutMax=[]  bOutMin=[]  bOutMax=[]  cOutMin=[]  cOutMax=[]  KbOutMin=[]  KbOutMax=[]  KtOutMin=[]  KtOutMax=[]  IntegratorOutMin=[]  IntegratorOutMax=[]  FilterOutMin=[]  FilterOutMax=[]  SumOutMin=[]  SumOutMax=[]  Sum1OutMin=[]  Sum1OutMax=[]  Sum2OutMin=[]  Sum2OutMax=[]  Sum3OutMin=[]  Sum3OutMax=[]  SumI1OutMin=[]  SumI1OutMax=[]  SumI2OutMin=[]  SumI2OutMax=[]  SumI3OutMin=[]  SumI3OutMax=[]  SumDOutMin=[]  SumDOutMax=[]  SaturationOutMin=[]  SaturationOutMax=[]  IntegratorContinuousStateAttributes=''  IntegratorStateMustResolveToSignalObject=off  IntegratorRTWStateStorageClass=Auto  FilterContinuousStateAttributes=''  FilterStateMustResolveToSignalObject=off  FilterRTWStateStorageClass=Auto  DifferentiatorICPrevScaledInput=0  DifferentiatorOutMin=[]  DifferentiatorOutMax=[]  FilterDiffOutCoefMin=[]  FilterDiffOutCoefMax=[]  SumDenOutMin=[]  SumDenOutMax=[]  SumNumOutMin=[]  SumNumOutMax=[]  ReciprocalOutMin=[]  ReciprocalOutMax=[]  DivideOutMin=[]  DivideOutMax=[]  TunerSelectOption=Transfer Function Based (PID Tuner App)
  cfblk6 : Gain  Gain=[-677144470.308883]
  cfblk7 : Sum  Inputs=+-
  cfblk8 : Subsystem
  cfblk9 : If  IfExpression=u1 >= 0  SampleTime=1
  cfblk2 : Outport
  wires:
  cfblk1/1 -> cfblk4/1
  cfblk11/1 -> cfblk7/1, cfblk12/4(cfblk17)
  cfblk12/1(cfblk2) -> cfblk8/1(cfblk1)
  cfblk13/1(cfblk2) -> cfblk7/2, cfblk5/2
  cfblk8/1(cfblk2) -> cfblk2/1, cfblk5/1, cfblk15/1
  cfblk4/1 -> cfblk6/1
  cfblk6/1 -> cfblk9/1, cfblk12/3(cfblk16)
  cfblk3/1 -> cfblk12/2(cfblk15)
  cfblk10/1 -> cfblk3/1
  cfblk9/1 -> cfblk12/Action
  cfblk9/2 -> cfblk13/Action
  cfblk5/1 -> cfblk14/1
  cfblk14/1 -> cfblk12/1(cfblk1)
  cfblk15/1 -> cfblk4/2
  cfblk7/1 -> cfblk16/1
  cfblk16/1 -> cfblk13/1(cfblk1)

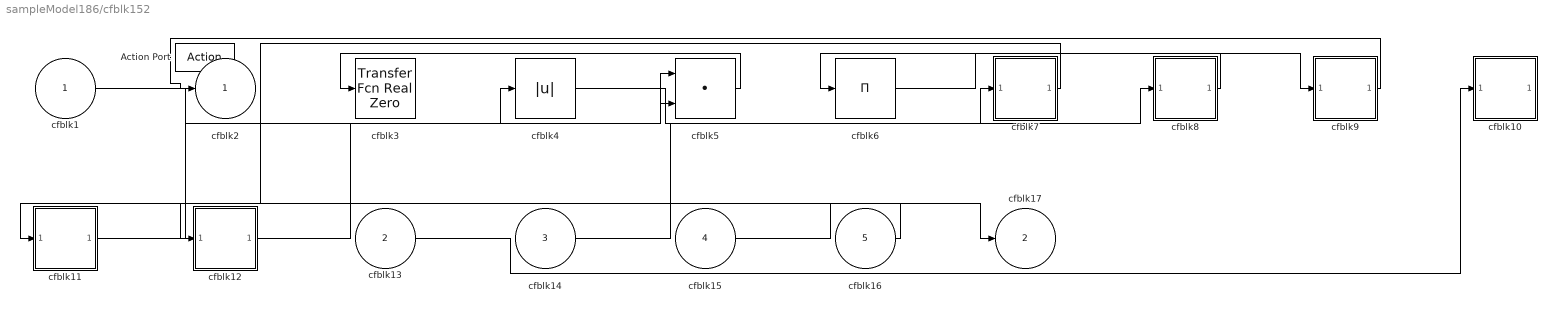
== system sampleModel186/cfblk152 ==
  cfblk1 : Inport
  cfblk13 : Inport  Port=2
  cfblk14 : Inport  Port=3
  cfblk15 : Inport  Port=4
  cfblk16 : Inport  Port=5
  Action Port : ActionPort  ActionType=else
  cfblk10 : Subsystem
  cfblk11 : Subsystem
  cfblk12 : Subsystem
  cfblk3 : simulink/Discrete/Transfer Fcn Real Zero  ZeroZ=0.75  ICPrevInput=0.0  DoSatur=off
      settings: SourceProductName=Simulink  SourceProductBaseCode=SL
  cfblk4 : Abs
  cfblk5 : DotProduct  InputSameDT=on  OutDataTypeStr=Inherit: Inherit via internal rule
  cfblk6 : Product  Inputs=*
  cfblk7 : Subsystem
  cfblk8 : Subsystem
  cfblk9 : Subsystem
  cfblk2 : Outport
  cfblk17 : Outport  Port=2
  wires:
  cfblk14/1 -> cfblk8/1(cfblk1)
  cfblk5/1 -> cfblk3/1
  cfblk7/1(cfblk2) -> cfblk11/1(cfblk1)
  cfblk12/1(cfblk2) -> cfblk5/1
  cfblk4/1 -> cfblk7/1(cfblk1)
  cfblk11/1(cfblk2) -> cfblk5/2
  cfblk13/1 -> cfblk10/1(cfblk1)
  cfblk1/1 -> cfblk4/1
  cfblk16/1 -> cfblk12/1(cfblk1)
  cfblk6/1 -> cfblk9/1(cfblk1)
  cfblk15/1 -> cfblk17/1
  cfblk9/1(cfblk2) -> cfblk2/1
  cfblk8/1(cfblk2) -> cfblk6/1

== system sampleModel186/cfblk153 ==
  cfblk1 : Inport
  cfblk9 : Inport  Port=2
  cfblk10 : Inport  Port=3
  cfblk11 : Inport  Port=4
  Action Port : ActionPort  ActionType=then
  cfblk13 : Delay
  cfblk3 : ComplexToRealImag
  cfblk4 : Subsystem
  cfblk5 : Subsystem
  cfblk6 : Subsystem
  cfblk7 : Subsystem
  cfblk8 : Subsystem
  cfblk2 : Outport
  cfblk12 : Outport  Port=2
  wires:
  cfblk10/1 -> cfblk6/1(cfblk1)
  cfblk11/1 -> cfblk5/1(cfblk1)
  cfblk8/1(cfblk2) -> cfblk2/1
  cfblk3/1 -> cfblk4/1(cfblk1)
  cfblk3/2 -> cfblk7/1(cfblk1)
  cfblk6/1(cfblk2) -> cfblk12/1
  cfblk9/1 -> cfblk8/1(cfblk1)
  cfblk7/1(cfblk2) -> cfblk13/1
  cfblk13/1 -> cfblk3/1

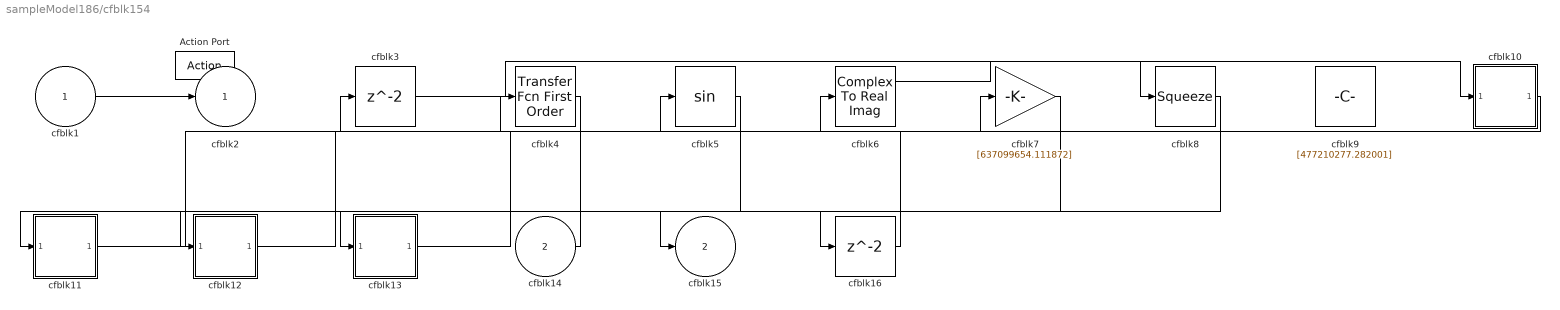
== system sampleModel186/cfblk154 ==
  cfblk1 : Inport
  cfblk14 : Inport  Port=2
  Action Port : ActionPort  ActionType=else
  cfblk10 : Subsystem
  cfblk11 : Subsystem
  cfblk12 : Subsystem
  cfblk13 : Subsystem
  cfblk16 : Delay
  cfblk3 : Delay
  cfblk4 : simulink/Discrete/Transfer Fcn First Order  PoleZ=0.95  ICPrevOutput=0.0  DoSatur=off
      settings: SourceProductName=Simulink
  cfblk5 : Trigonometry
  cfblk6 : ComplexToRealImag
  cfblk7 : Gain  Gain=[637099654.111872]
  cfblk8 : Squeeze
  cfblk9 : Constant  Value=[477210277.282001]  SampleTime=1
  cfblk2 : Outport
  cfblk15 : Outport  Port=2
  wires:
  cfblk3/1 -> cfblk8/1
  cfblk14/1 -> cfblk13/1(cfblk1)
  cfblk10/1(cfblk2) -> cfblk4/1
  cfblk4/1 -> cfblk11/1(cfblk1)
  cfblk12/1(cfblk2) -> cfblk5/1
  cfblk5/1 -> cfblk15/1
  cfblk11/1(cfblk2) -> cfblk7/1
  cfblk6/1 -> cfblk10/1(cfblk1)
  cfblk1/1 -> cfblk2/1
  cfblk13/1(cfblk2) -> cfblk6/1
  cfblk7/1 -> cfblk12/1(cfblk1)
  cfblk8/1 -> cfblk16/1
  cfblk16/1 -> cfblk3/1

== system sampleModel186/cfblk155 ==
  cfblk1 : Inport
  cfblk5 : Inport  Port=2
  Action Port : ActionPort  ActionType=then
  cfblk3 : Trigonometry
  cfblk4 : Subsystem
  cfblk2 : Outport
  cfblk6 : Outport  Port=2
  cfblk7 : Outport  Port=3
  wires:
  cfblk5/1 -> cfblk3/1, cfblk6/1
  cfblk4/1(cfblk2) -> cfblk7/1
  cfblk1/1 -> cfblk4/1(cfblk1)
  cfblk3/1 -> cfblk2/1

== system sampleModel186/cfblk156 ==
  cfblk1 : Inport
  cfblk11 : Inport  Port=2
  cfblk12 : Inport  Port=3
  cfblk13 : Inport  Port=4
  Action Port : ActionPort  ActionType=else
  cfblk10 : Subsystem
  cfblk3 : DiscreteStateSpace  SampleTime=-1
  cfblk4 : simulink/Discrete/Transfer Fcn Real Zero  ZeroZ=0.75  ICPrevInput=0.0  DoSatur=off
      settings: SourceProductName=Simulink  SourceProductBaseCode=SL
  cfblk5 : Sin  TimeSource=Use external signal  SampleTime=0
  cfblk6 : Constant  Value=[30460187.616230]  SampleTime=1
  cfblk7 : Subsystem
  cfblk8 : Subsystem
  cfblk9 : Subsystem
  cfblk2 : Outport
  wires:
  cfblk1/1 -> cfblk5/1
  cfblk4/1 -> cfblk2/1
  cfblk13/1 -> cfblk7/1(cfblk1)
  cfblk7/1(cfblk2) -> cfblk4/1
  cfblk12/1 -> cfblk10/1(cfblk1)
  cfblk6/1 -> cfblk3/1
  cfblk3/1 -> cfblk9/1(cfblk1)
  cfblk10/1(cfblk2) -> cfblk8/1(cfblk1)

== system sampleModel186/cfblk157 ==
  cfblk1 : Inport
  Action Port : ActionPort  ActionType=then
  cfblk3 : DiscreteTransferFcn
  cfblk4 : Constant  Value=[282260104.455071]  SampleTime=1
  cfblk5 : Subsystem
  cfblk6 : Subsystem
  cfblk7 : Subsystem
  cfblk2 : Outport
  wires:
  cfblk6/1(cfblk2) -> cfblk2/1
  cfblk5/1(cfblk2) -> cfblk3/1
  cfblk1/1 -> cfblk7/1(cfblk1)
  cfblk3/1 -> cfblk6/1(cfblk1)
  cfblk4/1 -> cfblk5/1(cfblk1)

== system sampleModel186/cfblk158 ==
  cfblk1 : Inport
  Action Port : ActionPort  ActionType=else
  cfblk10 : Subsystem
  cfblk11 : Subsystem
  cfblk12 : Subsystem
  cfblk13 : Delay
  cfblk3 : UnitDelay  SampleTime=-1
  cfblk4 : Sin  TimeSource=Use external signal  SampleTime=0
  cfblk5 : Sum  Inputs=+-
  cfblk6 : Constant  Value=[48957722.231244]  SampleTime=1
  cfblk7 : Constant  Value=[-200695089.141564]  SampleTime=1
  cfblk8 : Constant  Value=[-14995740.643667]  SampleTime=1
  cfblk9 : Subsystem
  cfblk2 : Outport
  wires:
  cfblk10/1(cfblk2) -> cfblk2/1
  cfblk12/1(cfblk2) -> cfblk4/1
  cfblk5/1 -> cfblk9/1(cfblk1)
  cfblk8/1 -> cfblk10/1(cfblk1)
  cfblk4/1 -> cfblk5/1
  cfblk1/1 -> cfblk11/1(cfblk1)
  cfblk11/1(cfblk2) -> cfblk12/1(cfblk1)
  cfblk6/1 -> cfblk3/1
  cfblk9/1(cfblk2) -> cfblk13/1
  cfblk13/1 -> cfblk5/2

== system sampleModel186/cfblk159 ==
  cfblk1 : Inport
  cfblk12 : Inport  Port=2
  Action Port : ActionPort  ActionType=then
  cfblk10 : Subsystem
  cfblk11 : Subsystem
  cfblk13 : Delay
  cfblk14 : Delay
  cfblk3 : simulink/Discrete/Tapped Delay  vinit=0.0  samptime=-1  NumDelays=1  DelayOrder=Oldest  includeCurrent=off
  cfblk4 : Rounding
  cfblk5 : PermuteDimensions
  cfblk6 : Sum  Inputs=+-
  cfblk7 : Assignment  DiagnosticForDimensions=Warning  IndexOptions=Index vector (dialog)  Indices=1  OutputSizes=1
  cfblk8 : Sum  Inputs=+
  cfblk9 : Subsystem
  cfblk2 : Outport
  wires:
  cfblk1/1 -> cfblk9/1(cfblk1)
  cfblk9/1(cfblk2) -> cfblk4/1
  cfblk12/1 -> cfblk2/1
  cfblk11/1(cfblk2) -> cfblk6/1
  cfblk3/1 -> cfblk7/1, cfblk7/2
  cfblk4/1 -> cfblk5/1
  cfblk6/1 -> cfblk10/1(cfblk1)
  cfblk5/1 -> cfblk8/1
  cfblk8/1 -> cfblk11/1(cfblk1)
  cfblk10/1(cfblk2) -> cfblk13/1
  cfblk13/1 -> cfblk6/2
  cfblk7/1 -> cfblk14/1
  cfblk14/1 -> cfblk3/1

== system sampleModel186/cfblk160 ==
  cfblk1 : Inport
  cfblk6 : Inport  Port=2
  Action Port : ActionPort  ActionType=else
  cfblk10 : Delay
  cfblk11 : Delay
  cfblk3 : Abs
  cfblk4 : Constant  Value=[199014671.579916]  SampleTime=1
  cfblk5 : If  IfExpression=u1 >= 0  SampleTime=1
  cfblk8 : Subsystem  TreatAsAtomicUnit=on
  cfblk9 : Subsystem  TreatAsAtomicUnit=on
  cfblk2 : Outport
  cfblk7 : Outport  Port=2
  wires:
  cfblk6/1 -> cfblk9/2(cfblk15)
  cfblk8/1(cfblk2) -> cfblk9/3(cfblk16)
  cfblk4/1 -> cfblk2/1, cfblk7/1
  cfblk1/1 -> cfblk8/1(cfblk1), cfblk8/2(cfblk12)
  cfblk8/2(cfblk13) -> cfblk3/1
  cfblk5/1 -> cfblk8/Action
  cfblk5/2 -> cfblk9/Action
  cfblk9/1(cfblk2) -> cfblk10/1
  cfblk10/1 -> cfblk5/1
  cfblk3/1 -> cfblk11/1
  cfblk11/1 -> cfblk9/1(cfblk1)

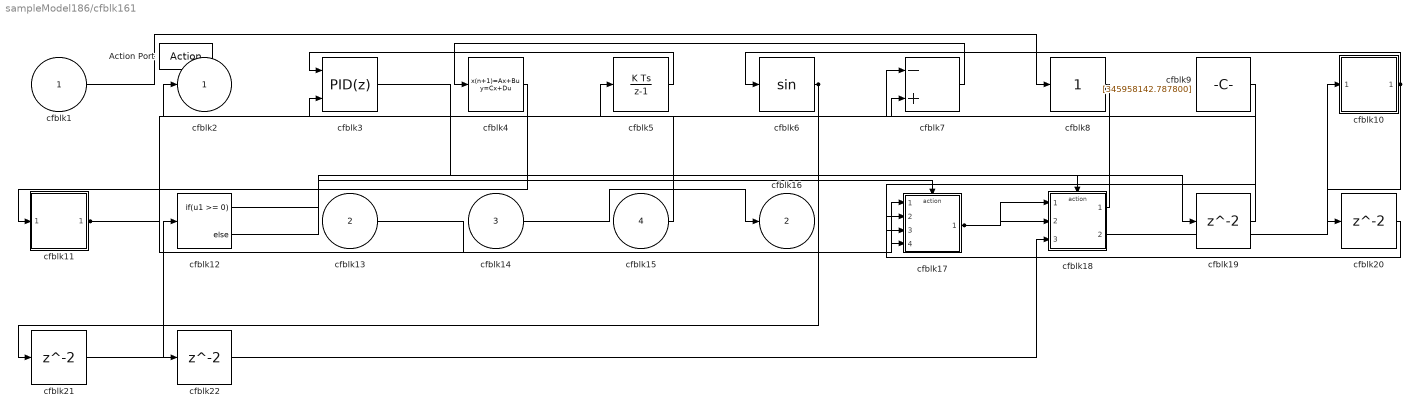
== system sampleModel186/cfblk161 ==
  cfblk1 : Inport
  cfblk13 : Inport  Port=2
  cfblk14 : Inport  Port=3
  cfblk15 : Inport  Port=4
  Action Port : ActionPort  ActionType=then
  cfblk10 : Subsystem
  cfblk11 : Subsystem
  cfblk12 : If  IfExpression=u1 >= 0  SampleTime=1
  cfblk17 : Subsystem  TreatAsAtomicUnit=on
  cfblk18 : Subsystem  TreatAsAtomicUnit=on
  cfblk{19..22} (4 alike) : Delay
  cfblk3 : simulink/Continuous/PID Controller (2DOF)  Controller=PID  TimeDomain=Discrete-time  SampleTime=-1  IntegratorMethod=Forward Euler  FilterMethod=Forward Euler  Form=Parallel  UseFilter=on  ControllerParametersSource=internal  P=1  I=1  D=0  N=100  b=1  c=1  InitialConditionSource=internal  InitialConditionForIntegrator=0  InitialConditionForFilter=0  ExternalReset=none  LimitOutput=off  UpperSaturationLimit=inf  LowerSaturationLimit=-inf  LinearizeAsGain=off  AntiWindupMode=none  Kb=1  TrackingMode=off  Kt=1  PParamMin=[]  PParamMax=[]  IParamMin=[]  IParamMax=[]  DParamMin=[]  DParamMax=[]  NParamMin=[]  NParamMax=[]  bParamMin=[]  bParamMax=[]  cParamMin=[]  cParamMax=[]  KbParamMin=[]  KbParamMax=[]  KtParamMin=[]  KtParamMax=[]  POutMin=[]  POutMax=[]  IOutMin=[]  IOutMax=[]  DOutMin=[]  DOutMax=[]  NOutMin=[]  NOutMax=[]  bOutMin=[]  bOutMax=[]  cOutMin=[]  cOutMax=[]  KbOutMin=[]  KbOutMax=[]  KtOutMin=[]  KtOutMax=[]  IntegratorOutMin=[]  IntegratorOutMax=[]  FilterOutMin=[]  FilterOutMax=[]  SumOutMin=[]  SumOutMax=[]  Sum1OutMin=[]  Sum1OutMax=[]  Sum2OutMin=[]  Sum2OutMax=[]  Sum3OutMin=[]  Sum3OutMax=[]  SumI1OutMin=[]  SumI1OutMax=[]  SumI2OutMin=[]  SumI2OutMax=[]  SumI3OutMin=[]  SumI3OutMax=[]  SumDOutMin=[]  SumDOutMax=[]  SaturationOutMin=[]  SaturationOutMax=[]  IntegratorContinuousStateAttributes=''  IntegratorStateMustResolveToSignalObject=off  IntegratorRTWStateStorageClass=Auto  FilterContinuousStateAttributes=''  FilterStateMustResolveToSignalObject=off  FilterRTWStateStorageClass=Auto  DifferentiatorICPrevScaledInput=0  DifferentiatorOutMin=[]  DifferentiatorOutMax=[]  FilterDiffOutCoefMin=[]  FilterDiffOutCoefMax=[]  SumDenOutMin=[]  SumDenOutMax=[]  SumNumOutMin=[]  SumNumOutMax=[]  ReciprocalOutMin=[]  ReciprocalOutMax=[]  DivideOutMin=[]  DivideOutMax=[]  TunerSelectOption=Transfer Function Based (PID Tuner App)
  cfblk4 : DiscreteStateSpace  SampleTime=-1
  cfblk5 : DiscreteIntegrator  SampleTime=-1  ICPrevOutput=DiscIntNeverNeededParam  ICPrevScaledInput=DiscIntNeverNeededParam
  cfblk6 : Trigonometry
  cfblk7 : Sum  Inputs=-+
  cfblk8 : simulink/Math Operations/Slider Gain  gain=1  low=0  high=2
  cfblk9 : Constant  Value=[345958142.787800]  SampleTime=1
  cfblk2 : Outport
  cfblk16 : Outport  Port=2
  wires:
  cfblk17/1(cfblk2) -> cfblk18/1(cfblk1), cfblk18/2(cfblk15)
  cfblk15/1 -> cfblk2/1
  cfblk7/1 -> cfblk4/1
  cfblk1/1 -> cfblk8/1
  cfblk13/1 -> cfblk17/1(cfblk1)
  cfblk4/1 -> cfblk11/1(cfblk1)
  cfblk18/1(cfblk2) -> cfblk5/1
  cfblk10/1(cfblk2) -> cfblk6/1, cfblk20/1
  cfblk18/2(cfblk17) -> cfblk10/1(cfblk1)
  cfblk8/1 -> cfblk7/2
  cfblk6/1 -> cfblk21/1, cfblk22/1
  cfblk9/1 -> cfblk17/3(cfblk10)
  cfblk11/1(cfblk2) -> cfblk17/4(cfblk11), cfblk3/2
  cfblk5/1 -> cfblk3/1
  cfblk14/1 -> cfblk16/1
  cfblk12/1 -> cfblk17/Action
  cfblk12/2 -> cfblk18/Action
  cfblk3/1 -> cfblk19/1
  cfblk19/1 -> cfblk7/1
  cfblk20/1 -> cfblk17/2(cfblk9)
  cfblk21/1 -> cfblk12/1
  cfblk22/1 -> cfblk18/3(cfblk16)

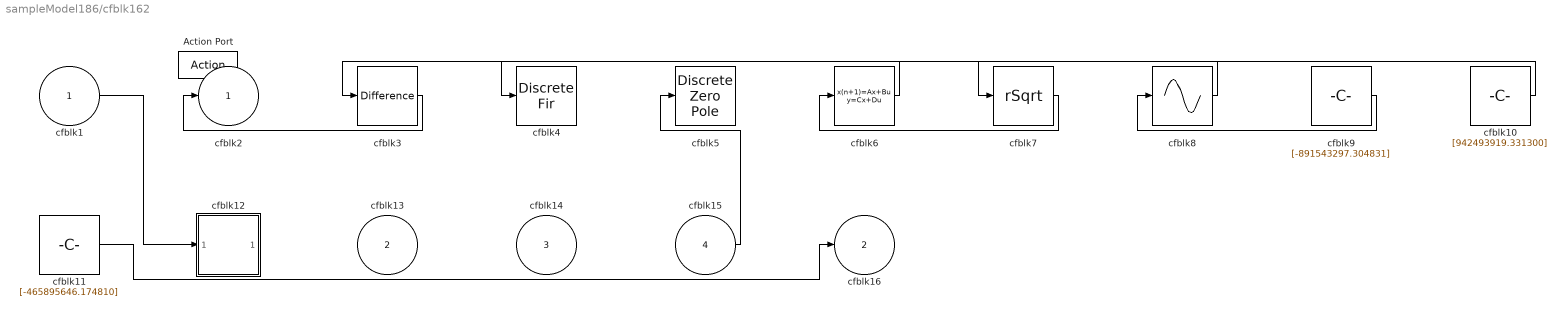
== system sampleModel186/cfblk162 ==
  cfblk1 : Inport
  cfblk13 : Inport  Port=2
  cfblk14 : Inport  Port=3
  cfblk15 : Inport  Port=4
  Action Port : ActionPort  ActionType=else
  cfblk10 : Constant  Value=[942493919.331300]  SampleTime=1
  cfblk11 : Constant  Value=[-465895646.174810]  SampleTime=1
  cfblk12 : Subsystem
  cfblk3 : simulink/Discrete/Difference  ICPrevInput=0.0  OutMin=[]  OutMax=[]  OutDataTypeStr=Inherit: Inherit via back propagation  OutDataType=fixdt(1, 16)  OutScaling=2^-10  DoSatur=off
  cfblk4 : DiscreteFir
  cfblk5 : DiscreteZeroPole  Poles=[0 0.5]  Gain=1  SampleTime=-1
  cfblk6 : DiscreteStateSpace  SampleTime=-1
  cfblk7 : Sqrt  Operator=rSqrt  AlgorithmType=Newton-Raphson  SaturateOnIntegerOverflow=on
  cfblk8 : Sin  TimeSource=Use external signal  SampleTime=0
  cfblk9 : Constant  Value=[-891543297.304831]  SampleTime=1
  cfblk2 : Outport
  cfblk16 : Outport  Port=2
  wires:
  cfblk15/1 -> cfblk5/1
  cfblk8/1 -> cfblk3/1
  cfblk7/1 -> cfblk6/1
  cfblk1/1 -> cfblk12/1(cfblk1)
  cfblk3/1 -> cfblk2/1
  cfblk11/1 -> cfblk16/1
  cfblk10/1 -> cfblk7/1
  cfblk6/1 -> cfblk4/1
  cfblk9/1 -> cfblk8/1

== system sampleModel186/cfblk147/cfblk13 ==
  cfblk1 : Inport
  cfblk8 : Inport  Port=2
  cfblk9 : Inport  Port=3
  cfblk10 : Inport  Port=4
  Action Port : ActionPort  ActionType=then
  cfblk11 : Delay
  cfblk3 : simulink/Discrete/Transfer Fcn Real Zero  ZeroZ=0.75  ICPrevInput=0.0  DoSatur=off
      settings: SourceProductName=Simulink  SourceProductBaseCode=SL
  cfblk4 : simulink/Discrete/Transfer Fcn Lead or Lag  PoleZ=0.95  ZeroZ=0.75  ICPrevOutput=0.0  ICPrevInput=0.0  DoSatur=off
      settings: SourceProductName=Simulink  SourceProductBaseCode=SL
  cfblk5 : ComplexToRealImag
  cfblk6 : Math  Operator=10^u  SaturateOnIntegerOverflow=on
  cfblk7 : Abs
  cfblk2 : Outport
  wires:
  cfblk10/1 -> cfblk7/1
  cfblk5/1 -> cfblk3/1
  cfblk5/2 -> cfblk6/1
  cfblk3/1 -> cfblk4/1
  cfblk4/1 -> cfblk2/1
  cfblk6/1 -> cfblk11/1
  cfblk11/1 -> cfblk5/1

== system sampleModel186/cfblk147/cfblk14 ==
  cfblk1 : Inport
  cfblk9 : Inport  Port=2
  cfblk10 : Inport  Port=3
  cfblk11 : Inport  Port=4
  cfblk12 : Inport  Port=5
  Action Port : ActionPort  ActionType=else
  cfblk3 : DiscreteFilter
  cfblk4 : ComplexToRealImag
  cfblk5 : ComplexToMagnitudeAngle
  cfblk6 : Constant  Value=[21050153.546396]  SampleTime=1
  cfblk7 : Subsystem
  cfblk8 : Subsystem
  cfblk2 : Outport
  cfblk13 : Outport  Port=2
  cfblk14 : Outport  Port=3
  wires:
  cfblk3/1 -> cfblk7/1(cfblk1)
  cfblk7/1(cfblk2) -> cfblk4/1
  cfblk10/1 -> cfblk2/1
  cfblk4/1 -> cfblk13/1
  cfblk12/1 -> cfblk14/1
  cfblk1/1 -> cfblk5/1
  cfblk5/1 -> cfblk3/1
  cfblk4/2 -> cfblk8/1(cfblk1)

== system sampleModel186/cfblk147/cfblk6 ==
  cfblk1 : Inport
  cfblk2 : Outport
  wires:
  cfblk1/1 -> cfblk2/1

== system sampleModel186/cfblk147/cfblk7 ==
  cfblk1 : Inport
  cfblk2 : Outport
  wires:
  cfblk1/1 -> cfblk2/1

== system sampleModel186/cfblk147/cfblk8 ==
  cfblk1 : Inport
  cfblk2 : Outport
  wires:
  cfblk1/1 -> cfblk2/1
